simulink model "Test"  (R2022a)
settings: Solver=VariableStepAuto  StartTime=0.0  StopTime=10.0  RelTol=1e-3
libraries: simulink x1
settings Model: Creator=Castiel  LastModifiedBy=Castiel

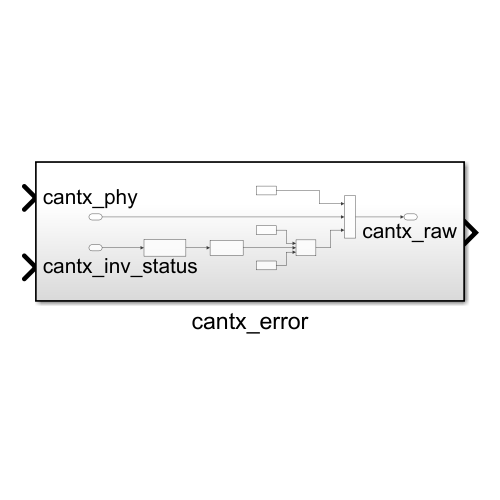
[thumbnail: Simulink's stored preview of the top-level diagram]
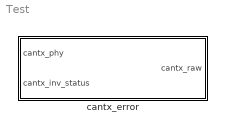
== system Test ==
  cantx_error : Subsystem

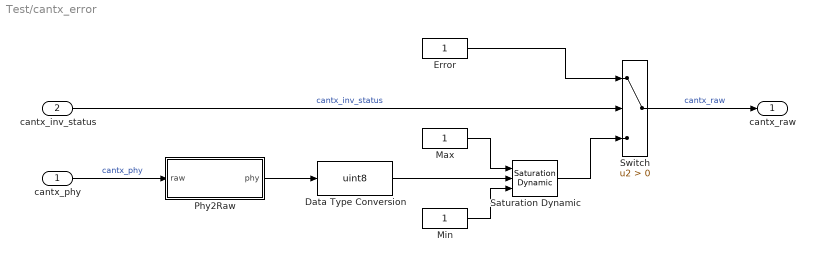
== system Test/cantx_error ==
  cantx_phy : Inport
  cantx_inv_status : Inport  Port=2
  Data Type Conversion : DataTypeConversion  OutDataTypeStr=uint8  SaturateOnIntegerOverflow=off  RndMeth=Floor
  Error : Constant
  Max : Constant
  Min : Constant
  Phy2Raw : Subsystem  mask{Offset=0, Factor=0}
      mask Callback Offset:
      | offset = get_param(gcb, 'Offset');
      |     set_param([gcb, '/Offset'], 'Value', offset);
      mask Callback Factor:
      | factor = get_param(gcb, 'Factor');
      |     set_param([gcb, '/Factor'], 'Value', factor);
      mask DialogControl DescGroupVar Prompt: Raw2Phy
      mask DialogControl ParameterGroupVar Prompt: 参数
      mask Display:
      | disp(['Offset = ', get_param(gcb, 'Offset'), '\n\n']);
      | disp(['Factor = ', get_param(gcb, 'Factor')]);
  Saturation Dynamic : simulink/Discontinuities/Saturation Dynamic  OutMin=[]  OutMax=[]  OutDataTypeStr=Inherit: Same as second input  OutDataType=fixdt(1, 16)  OutScaling=2^-10  DoSatur=off
  Switch : Switch  Criteria=u2 > Threshold  SaturateOnIntegerOverflow=off  InputSameDT=off
  cantx_raw : Outport
  wires:
  Switch/1 -> cantx_raw/1  "cantx_raw"
  Saturation Dynamic/1 -> Switch/3
  Phy2Raw/1(phy) -> Data Type Conversion/1
  Data Type Conversion/1 -> Saturation Dynamic/2
  cantx_phy/1 -> Phy2Raw/1(raw)  "cantx_phy"
  Min/1 -> Saturation Dynamic/3
  Error/1 -> Switch/1
  Max/1 -> Saturation Dynamic/1
  cantx_inv_status/1 -> Switch/2  "cantx_inv_status"

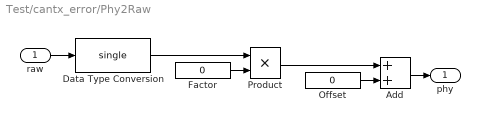
== system Test/cantx_error/Phy2Raw ==
  raw : Inport
  Add : Sum
  Data Type Conversion : DataTypeConversion  OutDataTypeStr=single  SaturateOnIntegerOverflow=off  RndMeth=Floor
  Factor : Constant  Value=0
  Offset : Constant  Value=0
  Product : Product
  phy : Outport
  wires:
  Add/1 -> phy/1
  Factor/1 -> Product/2
  Data Type Conversion/1 -> Product/1
  Offset/1 -> Add/2
  Product/1 -> Add/1
  raw/1 -> Data Type Conversion/1
